simulink model "prova"  (R2023a)
settings: Solver=VariableStepAuto  StartTime=0.0  StopTime=20  RelTol=1e-3
values from neighbouring files (symbols this model uses):
  A_lift = 3    [Main.m]    (also in SweepTest.m; myActiveSuspensions.mat)
  Cd_lift = 0.5    [Main.m]    (also in SweepTest.m; myActiveSuspensions.mat)
  DT = 1e-4    (= 0.0001)    [Main.m]    (also in SweepTest.m; myActiveSuspensions.mat)
  KS = K(:,1:n)    [Main.m]    (also in SweepTest.m; myActiveSuspensions.mat = [-6270.88767395 -1376.60013396 -1626.06750459 -11.6411551471)
  r0 = - g*ms/ks + l0s + Lift/ks    (= 0.603376724138)    [Main.m]    (also in SweepTest.m = 0.597040517241; myActiveSuspensions.mat = 0.597040517241)
  rho_lift = 1.225    [Main.m]    (also in SweepTest.m; myActiveSuspensions.mat)
  v = 10    [Main.m]    (also in SweepTest.m; myActiveSuspensions.mat)
  w0 = [d0; nu0; r0]    [Main.m]    (also in SweepTest.m; myActiveSuspensions.mat = [0 -91.875 0 0 0 0.597040517241])
  x_tilde_init = x_init - x0    [Main.m]    (also in SweepTest.m; myActiveSuspensions.mat = [0 0 0 0 0])
libraries: simulink x3
settings Model: Creator=loreb  LastModifiedBy=loreb

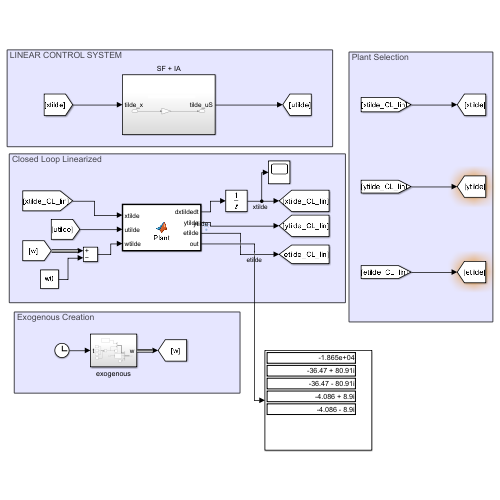
[thumbnail: Simulink's stored preview of the top-level diagram]
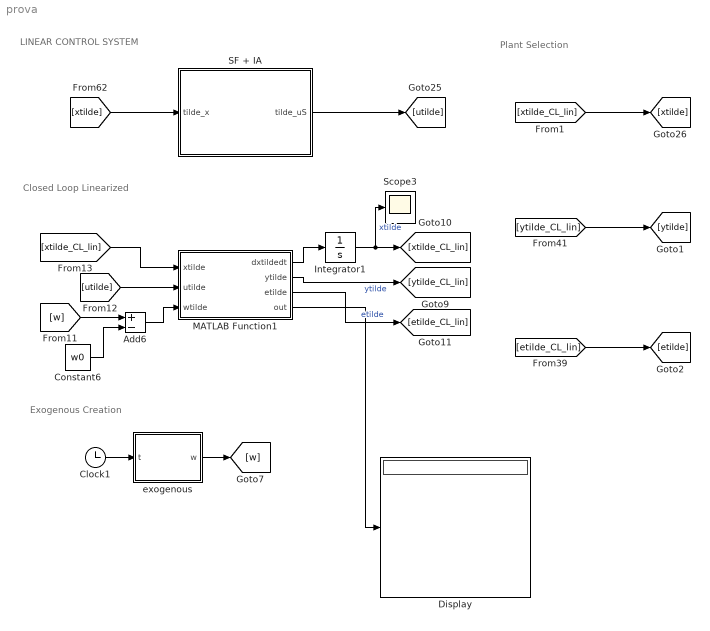
== system prova ==
  note: LINEAR CONTROL SYSTEM
  note: Closed Loop Linearized
  note: Exogenous Creation
  note: Plant Selection
  Add6 : Sum  Inputs=+-
  Clock1 : Clock
  Constant6 : Constant  Value=w0
  Display : Display
  Integrator1 : Integrator  InitialCondition=x_tilde_init
  MATLAB Function1 : MATLAB Function  TreatAsAtomicUnit=on
  SF + IA : Subsystem
  Scope3 : Scope
  exogenous : Subsystem
  wires:
  SF + IA/1(tilde_uS) -> [utilde]
  [xtilde] -> SF + IA/1(tilde_x)
  [xtilde_CL_lin] -> MATLAB Function1/1(xtilde)
  MATLAB Function1/2(ytilde) -> [ytilde_CL_lin]  "ytilde"
  Add6/1 -> MATLAB Function1/3(wtilde)
  [w] -> Add6/1
  MATLAB Function1/1(dxtildedt) -> Integrator1/1
  [utilde] -> MATLAB Function1/2(utilde)
  Integrator1/1 -> Scope3/1, [xtilde_CL_lin]  "xtilde"
  MATLAB Function1/3(etilde) -> [etilde_CL_lin]  "etilde"
  Constant6/1 -> Add6/2
  Clock1/1 -> exogenous/1(t)
  exogenous/1(w) -> [w]
  [etilde_CL_lin] -> [etilde]
  [xtilde_CL_lin] -> [xtilde]
  [ytilde_CL_lin] -> [ytilde]
  MATLAB Function1/4(out) -> Display/1

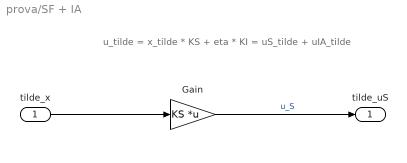
== system prova/SF + IA ==
  note: u_tilde = x_tilde * KS + eta * KI = uS_tilde + uIA_tilde
  tilde_x : Inport
  Gain : Gain  Gain=KS  Multiplication=Matrix(K*u)
  tilde_uS : Outport
  wires:
  Gain/1 -> tilde_uS/1  "u_S"
  tilde_x/1 -> Gain/1

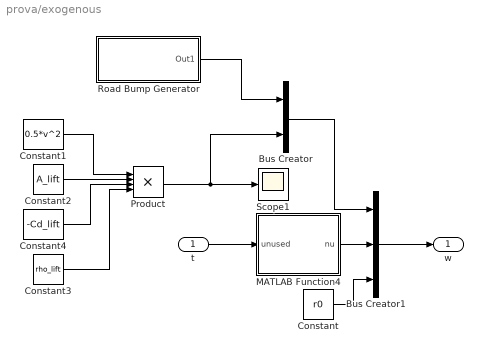
== system prova/exogenous ==
  t : Inport
  Bus Creator : BusCreator  Inputs=2
  Bus Creator1 : BusCreator  Inputs=3
  Constant : Constant  Value=r0
  Constant1 : Constant  Value=0.5*v^2  SampleTime=DT
  Constant2 : Constant  Value=A_lift  SampleTime=DT
  Constant3 : Constant  Value=rho_lift  SampleTime=DT
  Constant4 : Constant  Value=-Cd_lift  SampleTime=DT
  MATLAB Function4 : MATLAB Function  TreatAsAtomicUnit=on  SystemSampleTime=DT
  Product : Product  Inputs=4
  Road Bump Generator : Subsystem
  Scope1 : Scope
  w : Outport
  wires:
  Constant1/1 -> Product/1
  Road Bump Generator/1(Out1) -> Bus Creator/1
  Constant2/1 -> Product/2
  t/1 -> MATLAB Function4/1(unused)
  Constant3/1 -> Product/4
  Constant4/1 -> Product/3
  Product/1 -> Bus Creator/2, Scope1/1
  Bus Creator/1 -> Bus Creator1/1
  MATLAB Function4/1(nu) -> Bus Creator1/2
  Constant/1 -> Bus Creator1/3
  Bus Creator1/1 -> w/1

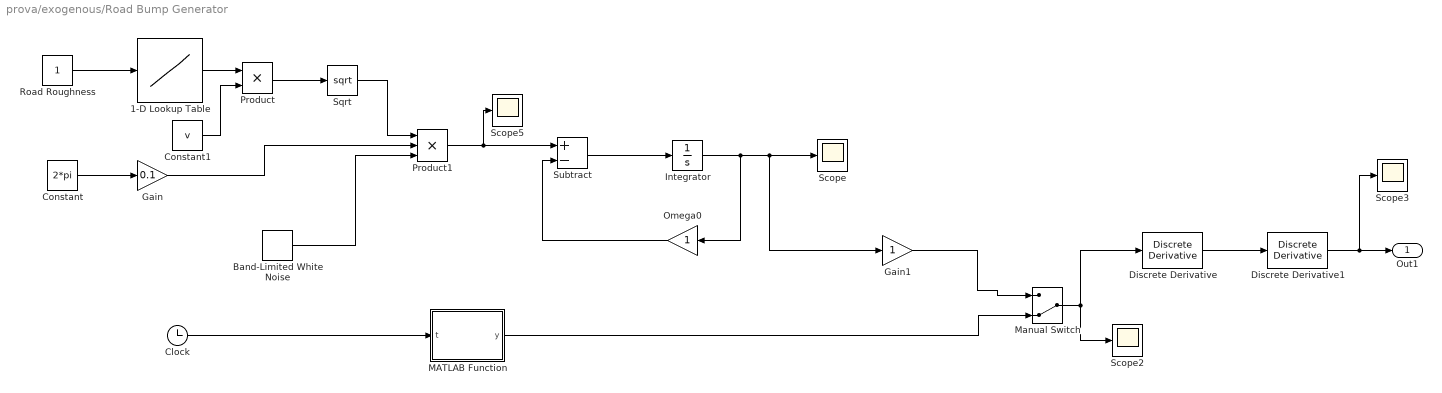
== system prova/exogenous/Road Bump Generator ==
  1-D Lookup Table : Lookup_n-D  NumberOfTableDimensions=1  BreakpointsForDimension1=[1;2;3;4;5;6;7;8]  Table=[1.6e-05;6.4e-05;0.000256;0.001024;0.004096;0.016384;0.065536;0.262144]  InternalRulePriority=Speed  RndMeth=Simplest
  Band-Limited White Noise : simulink/Sources/Band-Limited White Noise  Cov=0.1  Ts=0.01  seed=[23341]
  Clock : Clock
  Constant : Constant  Value=2*pi
  Constant1 : Constant  Value=v
  Discrete Derivative : simulink/Quick Insert/Discrete/Discrete Derivative  gainval=1.0  ICPrevScaledInput=0.0  OutMin=[]  OutMax=[]  OutDataType=fixdt(1, 16)  OutScaling=2^-10  DoSatur=off
  Discrete Derivative1 : simulink/Quick Insert/Discrete/Discrete Derivative  gainval=1.0  ICPrevScaledInput=0.0  OutMin=[]  OutMax=[]  OutDataType=fixdt(1, 16)  OutScaling=2^-10  DoSatur=off
  Gain : Gain  Gain=0.1
  Gain1 : Gain
  Integrator : Integrator
  MATLAB Function : MATLAB Function  TreatAsAtomicUnit=on
  Manual Switch : ManualSwitch  CurrentSetting=0
  Omega0 : Gain
  Product : Product
  Product1 : Product  Inputs=3
  Road Roughness : Constant
  Scope{,2..3,5} (4 alike) : Scope
  Sqrt : Sqrt
  Subtract : Sum  Inputs=+-
  Out1 : Outport
  wires:
  Subtract/1 -> Integrator/1
  Road Roughness/1 -> 1-D Lookup Table/1
  Clock/1 -> MATLAB Function/1(t)
  1-D Lookup Table/1 -> Product/1
  Sqrt/1 -> Product1/1
  Constant/1 -> Gain/1
  Band-Limited White Noise/1 -> Product1/3
  Omega0/1 -> Subtract/2
  MATLAB Function/1(y) -> Manual Switch/2
  Product1/1 -> Scope5/1, Subtract/1
  Integrator/1 -> Omega0/1, Gain1/1, Scope/1
  Constant1/1 -> Product/2
  Product/1 -> Sqrt/1
  Gain/1 -> Product1/2
  Gain1/1 -> Manual Switch/1
  Discrete Derivative/1 -> Discrete Derivative1/1
  Discrete Derivative1/1 -> Out1/1, Scope3/1
  Manual Switch/1 -> Scope2/1, Discrete Derivative/1

== matlab function prova/MATLAB Function1 ==
  data: xtilde input; utilde input; dxtildedt output; wtilde input; ytilde output; etilde output; out output
function [dxtildedt, ytilde, etilde,out] = Plant(xtilde,utilde,wtilde)

%% Plant Parameters
ks = 29000; % [N/m] spring coefficient
kt = 293000; % [N/m] tyre elastic coefficient
mu = 38;
ms = 295;
l0s = 0.7; % [m] lenght of the sprung for which the force is 0
l0t = 0.35; % [m]
g = 9.81;
betas = 3000; % damping coefficient 

A_lift = 3;
Cd_lift = 0.5; 
rho_lift = 1.225; %kg/m^3
v = 10; %[m/s] speed of the car
Lift = 0.5*A_lift*Cd_lift*(v^2)*rho_lift;

%% ACTUATOR PARAMETERS
beta = 1; %1/sec
mi = 1e-7; % scale coefficient to improve numerical conditioning of P
gamma = 1.545e9; % N/m^(5/2)kg^(1/2)
Ap = 3.35e-4; % m^2
Ps = 10342500; % Pa
alfa = 4.515e9; % N/m^5
rho = 865; % Kg/m^3 hydraulic fluid density found on internet

%% LINEARIZED MATRIXES

N = (ms+mu)/(ms*mu);

A = [0 1 0 0 0
    -ks*N -betas*N kt/mu 0 Ap/mi*N
    0 0 0 1 0
    ks/mu betas/mu -kt/mu 0 -Ap/(mu*mi)
    0 -mi*alfa*Ap 0 0 -beta];

B1 = [0;0;0;0;mi*gamma];

B2 = [0 0 0 0 0 0
    0 1/ms 0 0 0 0
    0 0 0 0 0 0
    -1 0 0 0 0 0
    0 0 0 0 0 0];

C = [1 0 0 0 0
    1 0 1 0 0
    -ks/ms -betas/ms 0 0 Ap/(mi*ms)];

D1 = [0;0;0];

D2 = [0 0 1 0 0 0
    0 0 0 1 0 0
    0 1/ms 0 0 1 0];

Ce = [1 0 0 0 0];  

De1 = 0;

De2 = [0 0 1 0 0 -1];

KS = [3.0928    9.6656    3.9963   -0.0002 -120.6763];
out=eig(A+B1*KS);
dxtildedt = A*xtilde+B1*utilde+B2*wtilde;
ytilde = C*xtilde+D1*utilde+D2*wtilde;
etilde = Ce*xtilde+De1*utilde+De2*wtilde;

== matlab function prova/exogenous/MATLAB Function4 ==
  data: unused input; nu output
function nu = noises(~)
std_pot = 0.001; % [m] potentiomenter standard deviation
std_laser = 0.001; %standard deviation laser
std_acc = 110e-6*sqrt(200); % [m/s^2] accelerometer standard deviation
nu = [std_pot*(2*rand(1)-1)
      std_laser*(2*rand(1)-1)
      std_acc*(2*rand(1)-1)];

end

== matlab function prova/exogenous/Road Bump Generator/MATLAB Function ==
  data: t input; y output
function y = fcn(t)

% Parameters definition

v = 10; % [m/s] speed of the vehicle

p = v*t; % [m] position that varies with time

pg = 50; % [m] pg is the position of the BEGINNING of the bump

l = 3; % [m] lenght of the hole/bump
h = 0.15; % [m] thickness of the hole/bump

lmat = [l^4 l^5 l^6 l^7 l^8; (l/2)^4 (l/2)^5 (l/2)^6 (l/2)^7 (l/2)^8; 4*l^3 5*l^4 6*l^5 7*l^6 8*l^7; 12*l^2 20*l^3 30*l^4 42*l^5 56*l^6; 24*l 60*l^2 120*l^3 210*l^4 336*l^5;];
lmatinv = inv(lmat);

cmat = zeros(5,1);
hmat = [0 h 0 0 0]';

cmat = lmatinv * hmat;

% Road profile function

if (p>pg && p-pg < l)
    sum = 0;
    for i = 0:8
        if i > 3
            sum = sum + cmat(i-3)*(p-pg)^(i);
        end
    end
    y = sum;
else
    y = 0;
end
